simulink model "Lab6"  (R2024b)
settings: Solver=ode8  StartTime=0.0  StopTime=10.0  FixedStep=0.01  RelTol=1e-3
values from neighbouring files (symbols this model uses):
  I = diag(Iv)    [initLab6.m]
  invI = inv(I)    [initLab6.m]
  w0 = [0; 0; 0]    [initLab6.m]
undefined symbols (not defined in the file or in its folder): env, IC
libraries: matrix_library x2
settings Model: Creator=filippocamaleonte  LastModifiedBy=elisa

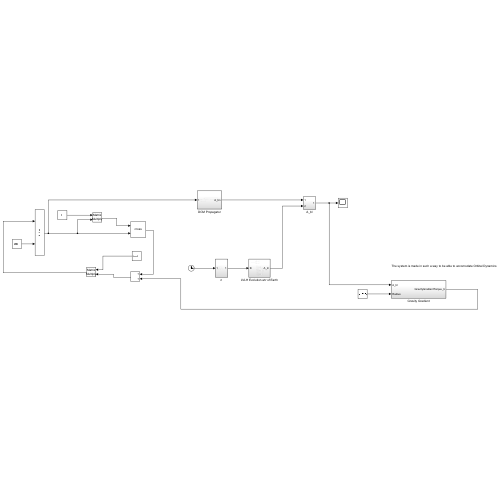
[thumbnail: Simulink's stored preview of the top-level diagram]
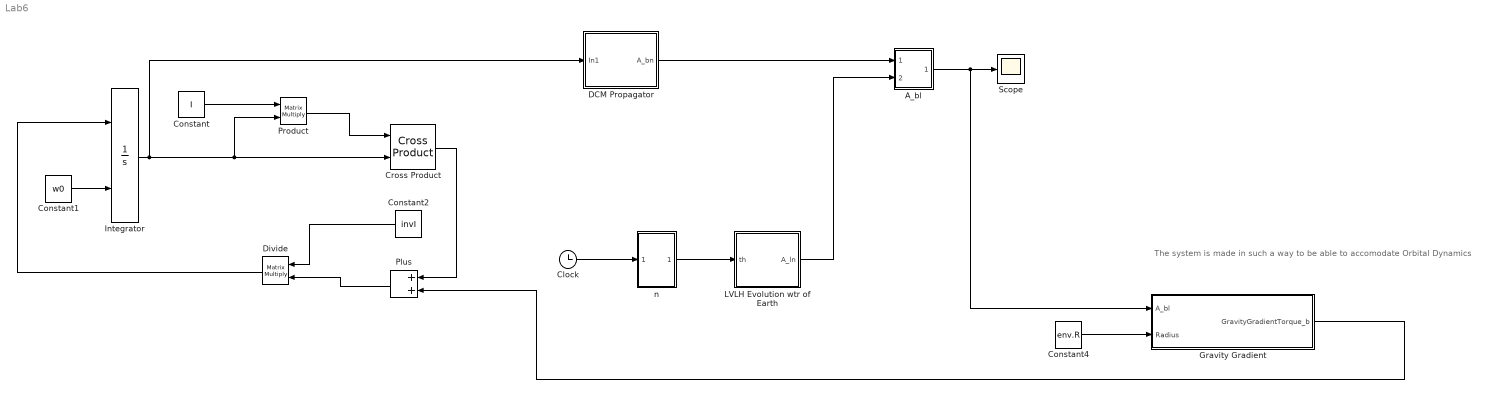
== system Lab6 ==
  note: The system is made in such a way to be able to accomodate Orbital Dynamics
  A_bl : Subsystem
  Clock : Clock
  Constant : Constant  Value=I
  Constant1 : Constant  Value=w0  VectorParams1D=off
  Constant2 : Constant  Value=invI
  Constant4 : Constant  Value=env.R
  Cross Product : matrix_library/Cross Product
  DCM Propagator : Subsystem
  Divide : Product  Inputs=**  Multiplication=Matrix(*)
  Gravity Gradient : Subsystem
  Integrator : Integrator  InitialConditionSource=external
  LVLH Evolution wtr of Earth : Subsystem
  Plus : Sum
  Product : Product  Multiplication=Matrix(*)
  Scope : Scope
  n : Subsystem
  wires:
  Divide/1 -> Integrator/1
  Product/1 -> Cross Product/1
  Cross Product/1 -> Plus/1
  Constant1/1 -> Integrator/2
  Integrator/1 -> DCM Propagator/1(In1), Product/2, Cross Product/2
  Constant2/1 -> Divide/1
  Constant/1 -> Product/1
  DCM Propagator/1(A_bn) -> A_bl/1(In1)
  LVLH Evolution wtr of Earth/1(A_ln) -> A_bl/2(In2)
  A_bl/1(Out1) -> Gravity Gradient/1(A_bl), Scope/1
  Clock/1 -> n/1(In1)
  n/1(Out1) -> LVLH Evolution wtr of Earth/1(th)
  Constant4/1 -> Gravity Gradient/2(Radius)
  Gravity Gradient/1(GravityGradientTorque_b) -> Plus/2
  Plus/1 -> Divide/2

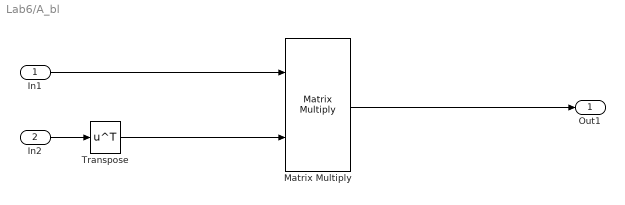
== system Lab6/A_bl ==
  In1 : Inport
  In2 : Inport  Port=2
  Matrix Multiply : Product  Multiplication=Matrix(*)
  Transpose : Math  Operator=transpose
  Out1 : Outport
  wires:
  Transpose/1 -> Matrix Multiply/2
  In2/1 -> Transpose/1
  Matrix Multiply/1 -> Out1/1
  In1/1 -> Matrix Multiply/1

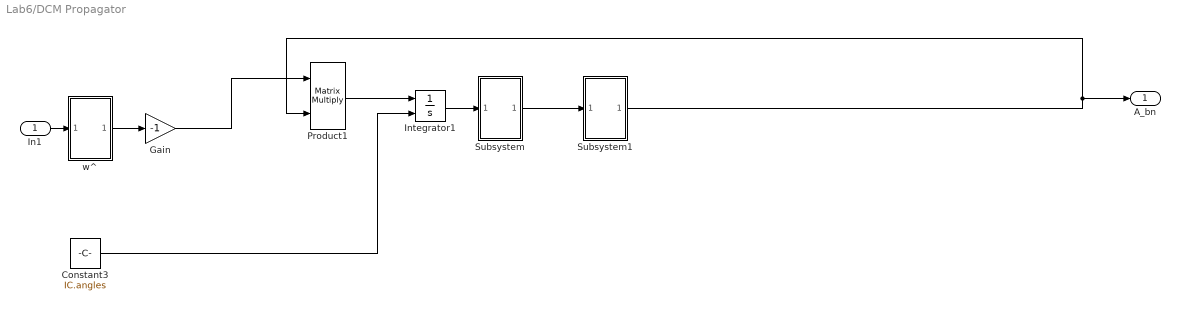
== system Lab6/DCM Propagator ==
  In1 : Inport
  Constant3 : Constant  Value=IC.angles
  Gain : Gain  Gain=-1
  Integrator1 : Integrator  InitialConditionSource=external
  Product1 : Product  Multiplication=Matrix(*)
  Subsystem : Subsystem
  Subsystem1 : Subsystem
  w^ : Subsystem
  A_bn : Outport
  wires:
  w^/1(Out1) -> Gain/1
  Gain/1 -> Product1/1
  In1/1 -> w^/1(In1)
  Product1/1 -> Integrator1/1
  Integrator1/1 -> Subsystem/1(In1)
  Subsystem/1(Out1) -> Subsystem1/1(In1)
  Constant3/1 -> Integrator1/2
  Subsystem1/1(Out1) -> Product1/2, A_bn/1

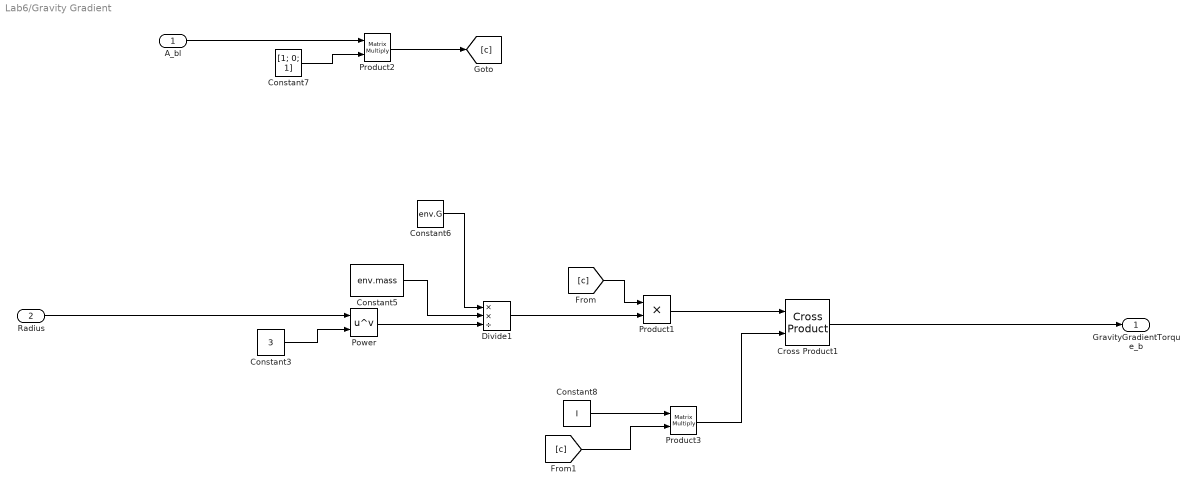
== system Lab6/Gravity Gradient ==
  A_bl : Inport
  Radius : Inport  Port=2
  Constant3 : Constant  Value=3
  Constant5 : Constant  Value=env.mass
  Constant6 : Constant  Value=env.G
  Constant7 : Constant  Value=[1; 0; 1]
  Constant8 : Constant  Value=I
  Cross Product1 : matrix_library/Cross Product
  Divide1 : Product  Inputs=**/
  Power : Math  Operator=pow
  Product1 : Product
  Product2 : Product  Multiplication=Matrix(*)
  Product3 : Product  Multiplication=Matrix(*)
  GravityGradientTorque_b : Outport
  wires:
  Divide1/1 -> Product1/2
  Power/1 -> Divide1/3
  Constant3/1 -> Power/2
  Constant7/1 -> Product2/2
  Radius/1 -> Power/1
  Constant5/1 -> Divide1/2
  Constant6/1 -> Divide1/1
  [c] -> Product3/2
  [c] -> Product1/1
  Product1/1 -> Cross Product1/1
  Cross Product1/1 -> GravityGradientTorque_b/1
  Constant8/1 -> Product3/1
  Product2/1 -> [c]
  Product3/1 -> Cross Product1/2
  A_bl/1 -> Product2/1

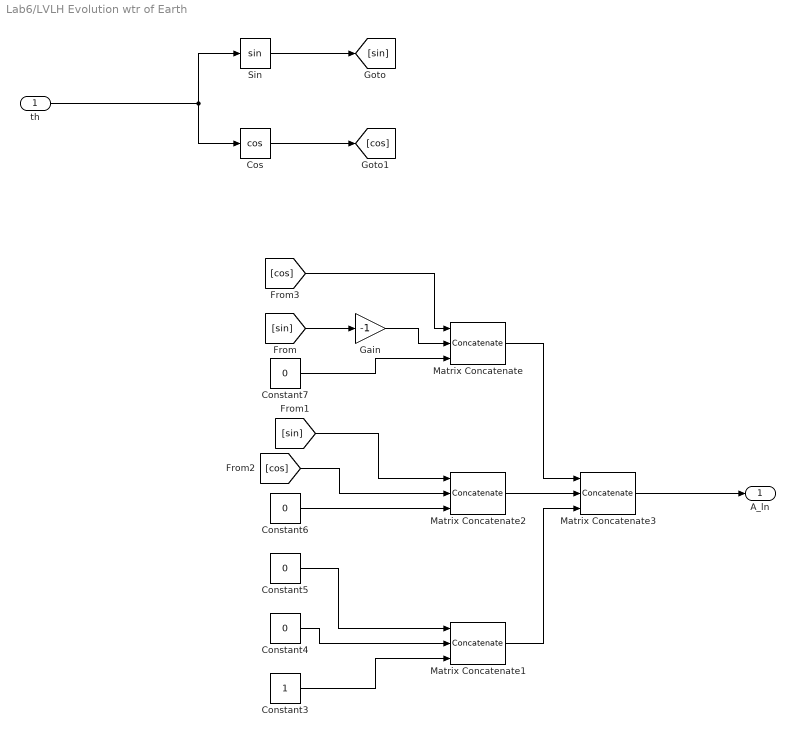
== system Lab6/LVLH Evolution wtr of Earth ==
  th : Inport
  Constant3 : Constant
  Constant{4..7} (4 alike) : Constant  Value=0
  Cos : Trigonometry  Operator=cos
  Gain : Gain  Gain=-1
  Matrix Concatenate : Concatenate  NumInputs=3  Mode=Multidimensional array
  Matrix Concatenate1 : Concatenate  NumInputs=3  Mode=Multidimensional array
  Matrix Concatenate2 : Concatenate  NumInputs=3  Mode=Multidimensional array
  Matrix Concatenate3 : Concatenate  NumInputs=3  Mode=Multidimensional array  ConcatenateDimension=2
  Sin : Trigonometry
  A_ln : Outport
  wires:
  Cos/1 -> [cos]
  Matrix Concatenate1/1 -> Matrix Concatenate3/3
  th/1 -> Cos/1, Sin/1
  Matrix Concatenate/1 -> Matrix Concatenate3/1
  Constant5/1 -> Matrix Concatenate1/1
  Constant3/1 -> Matrix Concatenate1/3
  [cos] -> Matrix Concatenate/1
  Sin/1 -> [sin]
  Constant6/1 -> Matrix Concatenate2/3
  Constant7/1 -> Matrix Concatenate/3
  Constant4/1 -> Matrix Concatenate1/2
  Matrix Concatenate2/1 -> Matrix Concatenate3/2
  [cos] -> Matrix Concatenate2/2
  [sin] -> Matrix Concatenate2/1
  Gain/1 -> Matrix Concatenate/2
  Matrix Concatenate3/1 -> A_ln/1
  [sin] -> Gain/1

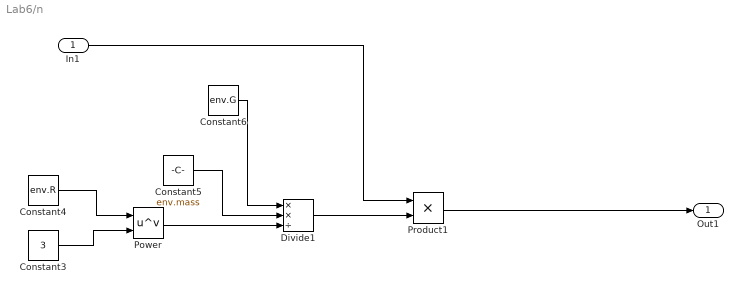
== system Lab6/n ==
  In1 : Inport
  Constant3 : Constant  Value=3
  Constant4 : Constant  Value=env.R
  Constant5 : Constant  Value=env.mass
  Constant6 : Constant  Value=env.G
  Divide1 : Product  Inputs=**/
  Power : Math  Operator=pow
  Product1 : Product
  Out1 : Outport
  wires:
  In1/1 -> Product1/1
  Divide1/1 -> Product1/2
  Constant6/1 -> Divide1/1
  Power/1 -> Divide1/3
  Constant5/1 -> Divide1/2
  Constant3/1 -> Power/2
  Product1/1 -> Out1/1
  Constant4/1 -> Power/1

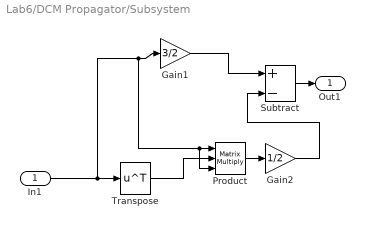
== system Lab6/DCM Propagator/Subsystem ==
  In1 : Inport
  Gain1 : Gain  Gain=3/2
  Gain2 : Gain  Gain=1/2
  Product : Product  Inputs=3  Multiplication=Matrix(*)
  Subtract : Sum  Inputs=+-
  Transpose : Math  Operator=transpose
  Out1 : Outport
  wires:
  In1/1 -> Product/3, Product/1, Gain1/1, Transpose/1
  Gain2/1 -> Subtract/2
  Gain1/1 -> Subtract/1
  Product/1 -> Gain2/1
  Transpose/1 -> Product/2
  Subtract/1 -> Out1/1

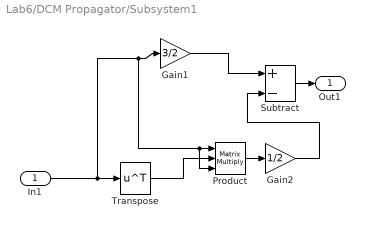
== system Lab6/DCM Propagator/Subsystem1 ==
  In1 : Inport
  Gain1 : Gain  Gain=3/2
  Gain2 : Gain  Gain=1/2
  Product : Product  Inputs=3  Multiplication=Matrix(*)
  Subtract : Sum  Inputs=+-
  Transpose : Math  Operator=transpose
  Out1 : Outport
  wires:
  In1/1 -> Product/3, Product/1, Gain1/1, Transpose/1
  Gain2/1 -> Subtract/2
  Gain1/1 -> Subtract/1
  Product/1 -> Gain2/1
  Transpose/1 -> Product/2
  Subtract/1 -> Out1/1

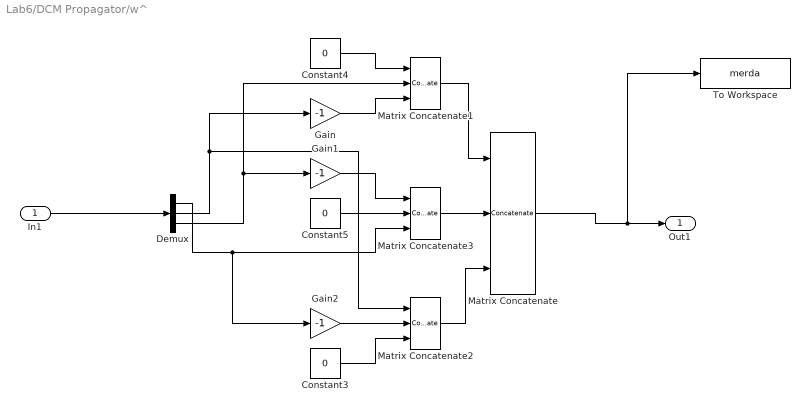
== system Lab6/DCM Propagator/w^ ==
  In1 : Inport
  Constant3 : Constant  Value=0
  Constant4 : Constant  Value=0
  Constant5 : Constant  Value=0
  Demux : Demux  Outputs=3
  Gain : Gain  Gain=-1
  Gain1 : Gain  Gain=-1
  Gain2 : Gain  Gain=-1
  Matrix Concatenate : Concatenate  NumInputs=3  Mode=Multidimensional array  ConcatenateDimension=2
  Matrix Concatenate1 : Concatenate  NumInputs=3  Mode=Multidimensional array
  Matrix Concatenate2 : Concatenate  NumInputs=3  Mode=Multidimensional array
  Matrix Concatenate3 : Concatenate  NumInputs=3  Mode=Multidimensional array
  To Workspace : ToWorkspace  VariableName=merda  SampleTime=-1
  Out1 : Outport
  wires:
  Demux/3 -> Gain1/1, Matrix Concatenate1/2
  Constant4/1 -> Matrix Concatenate1/1
  Matrix Concatenate/1 -> To Workspace/1, Out1/1
  Demux/1 -> Gain2/1, Matrix Concatenate3/3
  Constant5/1 -> Matrix Concatenate3/2
  Matrix Concatenate1/1 -> Matrix Concatenate/1
  Constant3/1 -> Matrix Concatenate2/3
  Matrix Concatenate2/1 -> Matrix Concatenate/3
  Matrix Concatenate3/1 -> Matrix Concatenate/2
  Gain2/1 -> Matrix Concatenate2/2
  Demux/2 -> Matrix Concatenate2/1, Gain/1
  Gain1/1 -> Matrix Concatenate3/1
  Gain/1 -> Matrix Concatenate1/3
  In1/1 -> Demux/1
